simulink model "Assignment1"  (R2016a)
settings: Solver=VariableStepAuto  StartTime=0.0  StopTime=10.0  RelTol=1e-3
libraries: hdlsllib x8
settings Model: Creator=duyvu  LastModifiedBy=duyvu

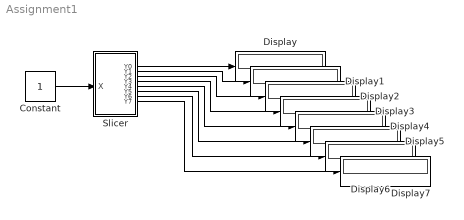
== system Assignment1 ==
  Constant : Constant  OutDataTypeStr=int8
  Display{,1..7} (8 alike) : Display
  Slicer : Subsystem
  wires:
  Constant/1 -> Slicer/1(X)
  Slicer/1("Y0 ") -> Display/1
  Slicer/2(Y1) -> Display1/1
  Slicer/3(Y2) -> Display2/1
  Slicer/4(Y3) -> Display3/1
  Slicer/5(Y4) -> Display4/1
  Slicer/6(Y5) -> Display5/1
  Slicer/7(Y6) -> Display6/1
  Slicer/8(Y7) -> Display7/1

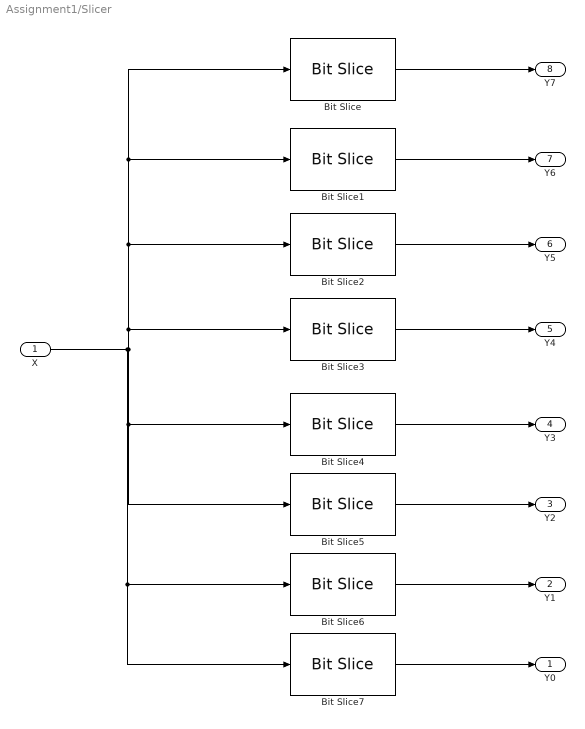
== system Assignment1/Slicer ==
  X : Inport  OutDataTypeStr=int8  SampleTime=1
  Bit Slice : hdlsllib/HDL Operations/Bit Slice  lidx=7  ridx=7
  Bit Slice1 : hdlsllib/HDL Operations/Bit Slice  lidx=6  ridx=6
  Bit Slice2 : hdlsllib/HDL Operations/Bit Slice  lidx=5  ridx=5
  Bit Slice3 : hdlsllib/HDL Operations/Bit Slice  lidx=4  ridx=4
  Bit Slice4 : hdlsllib/HDL Operations/Bit Slice  lidx=3  ridx=3
  Bit Slice5 : hdlsllib/HDL Operations/Bit Slice  lidx=2  ridx=2
  Bit Slice6 : hdlsllib/HDL Operations/Bit Slice  lidx=1  ridx=1
  Bit Slice7 : hdlsllib/HDL Operations/Bit Slice  lidx=0  ridx=0
  "Y0 " : Outport
  Y1 : Outport  Port=2
  Y2 : Outport  Port=3
  Y3 : Outport  Port=4
  Y4 : Outport  Port=5
  Y5 : Outport  Port=6
  Y6 : Outport  Port=7
  Y7 : Outport  Port=8
  wires:
  Bit Slice7/1 -> "Y0 "/1
  Bit Slice6/1 -> Y1/1
  Bit Slice3/1 -> Y4/1
  Bit Slice/1 -> Y7/1
  Bit Slice5/1 -> Y2/1
  Bit Slice4/1 -> Y3/1
  Bit Slice1/1 -> Y6/1
  Bit Slice2/1 -> Y5/1
  X/1 -> Bit Slice7/1, Bit Slice6/1, Bit Slice3/1, Bit Slice/1, Bit Slice1/1, Bit Slice2/1, Bit Slice4/1, Bit Slice5/1
